simulink model "ShipMPC_Optimal"  (R2020a)
settings: Solver=VariableStepAuto  StartTime=0.0  StopTime=tend  RelTol=1e-3
values from neighbouring files (symbols this model uses):
  tau_wave_amp = 0    [MPCobject.m]
  tau_wave_freq = 0    [MPCobject.m]
  Vc = 0    [MPCobject.m]
  Vref = 0.1    [MPCobject.m]
libraries: mpclib x2
settings Model: Creator=ahaseltalab  LastModifiedBy=localadmin
settings DataIOCC: ReturnWorkspaceOutputs=off
settings DebuggingCC: ArithmeticOperatorsInVariantConditions=warning
settings SFSimCC: SimUseLocalCustomCode=off  CustomCodeUndefinedFunction=UseInterfaceOnly
settings RTWCC: RTWUseLocalCustomCode=off
settings CodeAppCC: StateflowObjectComments=on

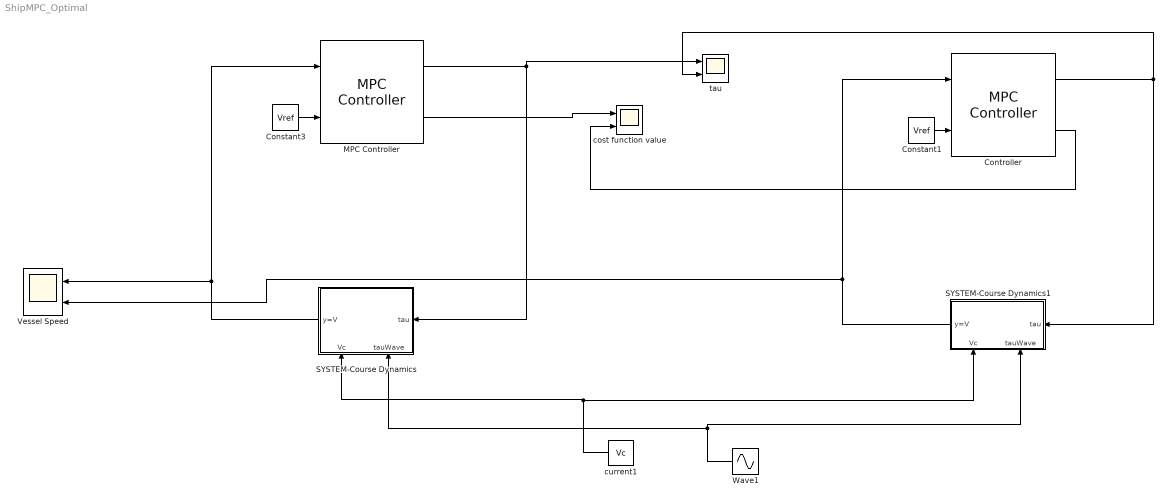
== system ShipMPC_Optimal ==
  " Wave1" : Sin  Amplitude=tau_wave_amp  Frequency=tau_wave_freq  SampleTime=0
  Constant1 : Constant  Value=Vref
  Constant3 : Constant  Value=Vref
  Controller : mpclib/MPC Controller  SCDEnableBlockLinearizationSpecification=on  mpcobj=MPCobj2  is_multiple=0  enable_value=0  return_u0=off  updateMPCinCallerWorkspace=on  md_inport=off  mv_inport=off  uref_inport=off  return_cost=on  return_mvseq=off  return_qpstatus=off  return_xseq=off  return_state=off  return_ovseq=off  state_inport=off  umin_inport=off  umax_inport=off  ymin_inport=off  ymax_inport=off  cc_inport=off  ywt_inport=off  uwt_inport=off  duwt_inport=off  rhoeps_inport=off  pm_inport=off  MaximumP=10  HorizonChoice=FixedHorizon  n_ts=1  n_p=100  n_mv=1  n_md=0  n_ud=0  n_mo=1  n_uo=0  BlockDataType=double  SampleTimeInherited=off  switch_inport=off
  MPC Controller : mpclib/MPC Controller  SCDEnableBlockLinearizationSpecification=on  mpcobj=MPCobj  is_multiple=0  enable_value=0  return_u0=off  updateMPCinCallerWorkspace=on  md_inport=off  mv_inport=off  uref_inport=off  return_cost=on  return_mvseq=off  return_qpstatus=off  return_xseq=off  return_state=off  return_ovseq=off  state_inport=off  umin_inport=off  umax_inport=off  ymin_inport=off  ymax_inport=off  cc_inport=off  ywt_inport=off  uwt_inport=off  duwt_inport=off  rhoeps_inport=off  pm_inport=off  MaximumP=10  HorizonChoice=FixedHorizon  n_ts=1  n_p=20  n_mv=1  n_md=0  n_ud=0  n_mo=1  n_uo=0  BlockDataType=double  SampleTimeInherited=off  switch_inport=off
  SYSTEM-Course Dynamics : Subsystem
      settings: PortSchema="{\"entries\":[{\"content\":{\"sides\":[{\"content\":{\"connectorIds\":[\"In1\"]},\"type\":\"ConnectorPlacement.EquallySpacedRectSide\",\"uuid\":\"4f22bad8-6928-4451-9730-7c1f78fa808f\"},{\"content\":{\"connectorIds\":[\"Out1\"],\"side\":\"RIGHT\"},\"type\":\"ConnectorPlacement.EquallySpacedRectSide\",\"uuid\":\"85a58395-212e-4d16-a9c9-4f5aadeccab2\"},{\"content\":{\"connectorIds\":[],\"side\":\"TOP\"},\"type\":\"ConnectorPlacement.EquallySpacedRectSide\",\"uuid\":\"d0f348e3-7d39-4292-8f6d-ffa1719d3969\"},{\"content\":{\"connectorIds\":[\"In2\",\"In3\"],\"side\":\"BOTTOM\"},\"type\":\"ConnectorPlacement.EquallySpacedRectSide\",\"uuid\":\"664e988f-132c-4835-9901-30573651760b\"}]},\"type\":\"ConnectorPlacement.EquallySpacedConnector\",\"uuid\":\"020c6d9a-4c68-4a1d-9c74-9250f81b52b7\"}],\"packageUris\":[\"http://schema.mathworks.com/mf0/Connector/19700101\"],\"version\":\"1.0\"}"
  SYSTEM-Course Dynamics1 : Subsystem
      settings: PortSchema="{\"entries\":[{\"content\":{\"sides\":[{\"content\":{\"connectorIds\":[\"In1\"]},\"type\":\"ConnectorPlacement.EquallySpacedRectSide\",\"uuid\":\"4f22bad8-6928-4451-9730-7c1f78fa808f\"},{\"content\":{\"connectorIds\":[\"Out1\"],\"side\":\"RIGHT\"},\"type\":\"ConnectorPlacement.EquallySpacedRectSide\",\"uuid\":\"85a58395-212e-4d16-a9c9-4f5aadeccab2\"},{\"content\":{\"connectorIds\":[],\"side\":\"TOP\"},\"type\":\"ConnectorPlacement.EquallySpacedRectSide\",\"uuid\":\"d0f348e3-7d39-4292-8f6d-ffa1719d3969\"},{\"content\":{\"connectorIds\":[\"In2\",\"In3\"],\"side\":\"BOTTOM\"},\"type\":\"ConnectorPlacement.EquallySpacedRectSide\",\"uuid\":\"013912bf-dea1-4c74-9fca-9f9c221613e4\"}]},\"type\":\"ConnectorPlacement.EquallySpacedConnector\",\"uuid\":\"020c6d9a-4c68-4a1d-9c74-9250f81b52b7\"}],\"packageUris\":[\"http://schema.mathworks.com/mf0/Connector/19700101\"],\"version\":\"1.0\"}"
  Vessel Speed : Scope  NumInputPorts=2
  cost function value : Scope  NumInputPorts=2
  current1 : Constant  Value=Vc
  tau : Scope  NumInputPorts=2
  wires:
  MPC Controller/1 -> tau/1, SYSTEM-Course Dynamics/1(tau)
  MPC Controller/2 -> cost function value/1
  SYSTEM-Course Dynamics/1(y=V) -> MPC Controller/1, Vessel Speed/1
  " Wave1"/1 -> SYSTEM-Course Dynamics/2(tauWave), SYSTEM-Course Dynamics1/2(tauWave)
  current1/1 -> SYSTEM-Course Dynamics/3(Vc), SYSTEM-Course Dynamics1/3(Vc)
  Constant1/1 -> Controller/2
  SYSTEM-Course Dynamics1/1(y=V) -> Vessel Speed/2, Controller/1
  Controller/1 -> tau/2, SYSTEM-Course Dynamics1/1(tau)
  Controller/2 -> cost function value/2
  Constant3/1 -> MPC Controller/2

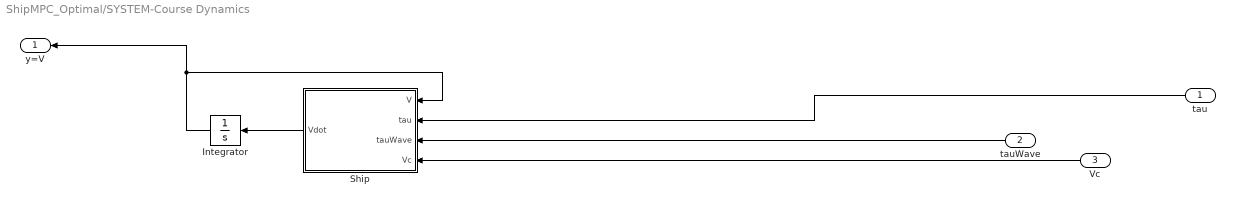
== system ShipMPC_Optimal/SYSTEM-Course Dynamics ==
  tau : Inport
  tauWave : Inport  Port=2
  Vc : Inport  Port=3
  Integrator : Integrator
  Ship : MATLAB Function  TreatAsAtomicUnit=on
  y=V : Outport
  wires:
  Vc/1 -> Ship/4(Vc)
  tauWave/1 -> Ship/3(tauWave)
  tau/1 -> Ship/2(tau)
  Ship/1(Vdot) -> Integrator/1
  Integrator/1 -> y=V/1, Ship/1(V)

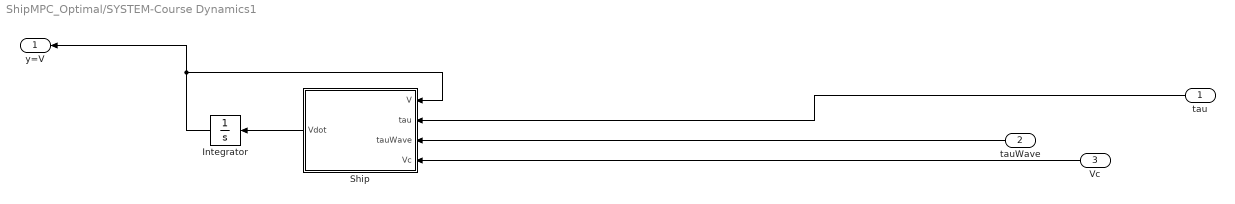
== system ShipMPC_Optimal/SYSTEM-Course Dynamics1 ==
  tau : Inport
  tauWave : Inport  Port=2
  Vc : Inport  Port=3
  Integrator : Integrator
  Ship : MATLAB Function  TreatAsAtomicUnit=on
  y=V : Outport
  wires:
  Vc/1 -> Ship/4(Vc)
  tauWave/1 -> Ship/3(tauWave)
  tau/1 -> Ship/2(tau)
  Ship/1(Vdot) -> Integrator/1
  Integrator/1 -> y=V/1, Ship/1(V)

== matlab function ShipMPC_Optimal/SYSTEM-Course Dynamics1/Ship ==
  data: V input; Vdot output; tau input; tauWave input; Vc input
function Vdot = fcn(V,tau,tauWave,Vc)

m=23.8;
ma=2;

Rs=-1.44;


Vdot = (1/(m+ma))*(Rs*(V-Vc)+tau+tauWave);

== matlab function ShipMPC_Optimal/SYSTEM-Course Dynamics/Ship ==
  data: V input; Vdot output; tau input; tauWave input; Vc input
function Vdot = fcn(V,tau,tauWave,Vc)

m=23.8;
ma=2;

Rs=-1.44;


Vdot = (1/(m+ma))*(Rs*(V-Vc)+tau+tauWave);
